simulink model "DC_motor_control"  (Simulink 7.2)
settings: Solver=ode23s  StartTime=0.0  StopTime=5  RelTol=1e-3
libraries: powerlib x6, simulink x2
settings Model: Creator=ahmed-salah  LastModifiedBy=ahmed-salah
settings SolverCC: ZeroCrossAlgorithm=Adaptive

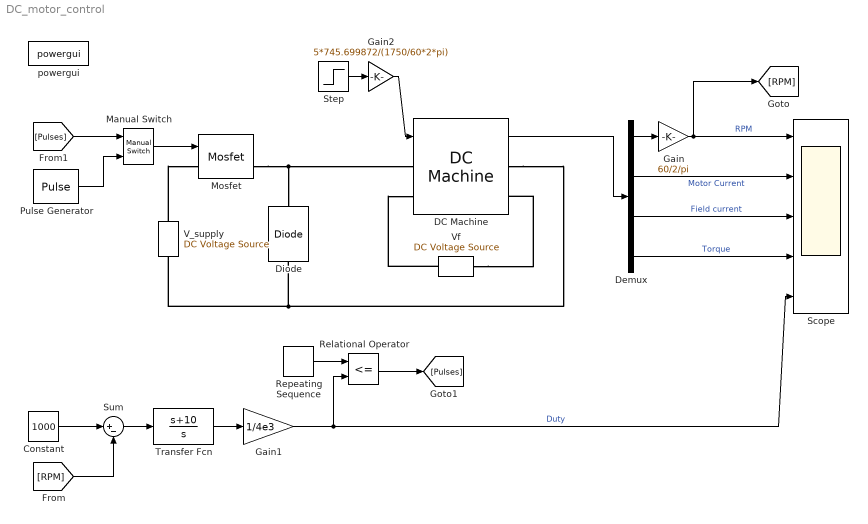
== system DC_motor_control ==
  Constant : Constant  Value=1000  OutDataType=sfix(16)  OutScaling=2^0
  DC Machine : powerlib/Machines/DC Machine  DialogController=POWERSYS.PowerSysDialog  SystemSampleTime=-1  PresetModel=01: 5HP 240V 1750RPM Field:300V  MechanicalLoad=Torque TL  ShowDetailedParameters=on  RLa=[2.581 0.028]  RLf=[281.3 156]  Laf=0.9483  J=0.02215  Bm=0.002953  Tf=0.5161  w0=0  Ifinit=0.53323853537149  TsPowergui=0  TsBlock=-1
  Demux : Demux
  Diode : powerlib/Power Electronics/Diode  Orientation=up  DialogController=POWERSYS.PowerSysDialog  SystemSampleTime=-1  Ron=0.001  Lon=0  Vf=0.8  IC=0  UseSnubber=off  Rs=500  Cs=250e-9  Measurements=off
  Gain : Gain  Gain=60/2/pi  ParameterDataType=sfix(16)  ParameterScaling=2^0  OutDataType=sfix(16)  OutScaling=2^0
  Gain1 : Gain  Gain=1/4e3  ParameterDataType=sfix(16)  ParameterScaling=2^0  OutDataType=sfix(16)  OutScaling=2^0
  Gain2 : Gain  Gain=5*745.699872/(1750/60*2*pi)  ParameterDataType=sfix(16)  ParameterScaling=2^0  OutDataType=sfix(16)  OutScaling=2^0
  Manual Switch : simulink/Signal Routing/Manual Switch  SystemSampleTime=-1  sw=1  action=0  varsize=off
  Mosfet : powerlib/Power Electronics/Mosfet  DialogController=POWERSYS.PowerSysDialog  SystemSampleTime=-1  Ron=0.1  Lon=0  Rd=0.01  Vfd=0  IC=0  Rs=1e5  Cs=inf  Measurements=on
  Pulse Generator : DiscretePulseGenerator  PulseType=Time based  Amplitude=100  Period=1/1e3  PulseWidth=30
  Relational Operator : RelationalOperator  Operator=<=  LogicOutDataTypeMode=boolean  OutDataTypeStr=boolean  SampleTime=0
  Repeating Sequence : simulink/Sources/Repeating Sequence  SystemSampleTime=-1  rep_seq_t=[0 1 ]/1e3  rep_seq_y=[0 1 ]
  Scope : Scope  NumInputPorts=5
      settings: TimeRange=5  YMin=-250~0~0.506577~0~0.2  YMax=1500~40~0.559901~20~0.475
  Step : Step  Time=2.5  Before=.1  After=0.7  SampleTime=0
  Sum : Sum  Inputs=|+-  OutDataType=sfix(16)  OutScaling=2^0
  Transfer Fcn : TransferFcn  Numerator=[1 10]  Denominator=[1 0]
  V_supply : powerlib/Electrical Sources/DC Voltage Source  Orientation=up  DialogController=POWERSYS.PowerSysDialog  SystemSampleTime=-1  Amplitude=300  Measurements=None
  Vf : powerlib/Electrical Sources/DC Voltage Source  Orientation=left  DialogController=POWERSYS.PowerSysDialog  SystemSampleTime=-1  Amplitude=150  Measurements=None
  powergui : powerlib/powergui  SystemSampleTime=-1  SimulationMode=Continuous  SampleTime=50e-6  frequency=60  SPID=off  DisableSnubberDevices=off  DisableRonSwitches=off  DisableVfSwitches=off  SwTol=0  Interpol=off  frequencyindice=0  echomessages=off  HookPort=off  FunctionMessages=off  EnableUseOfTLC=off  x0status=blocks  RestoreLinks=warning  Frange=[0:2:500]  Ylog=off  Xlog=on  ShowGrid=off  save=off  variable=ZData  ZoomFFT=on  StartTime=0.0  cycles=1  DisplayStyle=1  fundamental=60  FreqAxis=off  MaxFrequency=1000  frequencyindicesteady=1  RmsSteady=1  display=off  Ts=0  methode=off
  wires:
  DC Machine/1 -> Demux/1
  Step/1 -> Gain2/1
  Demux/1 -> Gain/1
  Demux/2 -> Scope/2  "Motor Current"
  Demux/3 -> Scope/3  "Field current"
  Gain/1 -> [RPM], Scope/1  "RPM"
  Gain1/1 -> Relational Operator/2, Scope/5  "Duty"
  Repeating Sequence/1 -> Relational Operator/1
  Constant/1 -> Sum/1
  Sum/1 -> Transfer Fcn/1
  Transfer Fcn/1 -> Gain1/1
  Relational Operator/1 -> [Pulses]
  Gain2/1 -> DC Machine/1
  [RPM] -> Sum/2
  Manual Switch/1 -> Mosfet/1
  [Pulses] -> Manual Switch/1
  Pulse Generator/1 -> Manual Switch/2
  Demux/4 -> Scope/4  "Torque"
  connections:
  Vf/RConn1 -- DC Machine/LConn2
  Vf/LConn1 -- DC Machine/RConn2
  V_supply/RConn1 -- Mosfet/LConn1
  DC Machine/RConn1 -- V_supply/LConn1 -- Diode/LConn1
  Mosfet/RConn1 -- DC Machine/LConn1 -- Diode/RConn1
